simulink model "MORUS_NELINEARNI_NELINEARNI_MPC_2"  (R2019a)
settings: Solver=FixedStepAuto  StartTime=0.0  StopTime=sim_time  RelTol=1e-3  EnableMultiTasking=on
values from neighbouring files (symbols this model uses):
  A_dis_calc = expm(kSamplingTime*A_continous_time)    [MPC_designer_X.m]    (also in NonTilting.m; RUN_simulation.m; Simulacija_MPC_YAW_NELINEARNI.m; Simulacija_MPC_Z.m)
  B_dis_calc = integral_exp_A * B_continous_time    [MPC_designer_X.m]    (also in NonTilting.m; RUN_simulation.m; Simulacija_MPC_YAW_NELINEARNI.m; Simulacija_MPC_Z.m)
  b_f = 4.56e-4    (= 0.000456)    [LinearizacijaMatrica.m]    (also in Linearizirane_matrice.mat; MPC_designer_X.m; NonTilting.m; RUN_simulation.m)
  b_m = 0.01    [LinearizacijaMatrica.m]    (also in Linearizirane_matrice.mat; MPC_designer_X.m; NonTilting.m; RUN_simulation.m)
  BETA = 0.0    (= 0)    [LinearizacijaMatrica.m]    (also in Linearizirane_matrice.mat; MPC_designer_X.m; NonTilting.m = 0.200712863979; RUN_simulation.m)
  g = 9.80665    [LinearizacijaMatrica.m]    (also in Linearizirane_matrice.mat; MPC_designer_X.m = 9.81; NonTilting.m = 9.81; RUN_simulation.m = 9.81)
  hover = 427.6233    [MPC_designer_X.m]    (also in NonTilting.m; RUN_simulation.m; Simulacija_MPC_YAW_NELINEARNI.m; Simulacija_MPC_Z.m)
  I_b_xx = 5.5268    [MPC_designer_X.m]    (also in NonTilting.m; RUN_simulation.m; Simulacija_MPC_YAW_NELINEARNI.m; Simulacija_MPC_Z.m)
  I_b_yy = 5.5268    [MPC_designer_X.m]    (also in NonTilting.m; RUN_simulation.m; Simulacija_MPC_YAW_NELINEARNI.m; Simulacija_MPC_Z.m)
  I_b_zz = 6.8854    [MPC_designer_X.m]    (also in NonTilting.m; RUN_simulation.m; Simulacija_MPC_YAW_NELINEARNI.m; Simulacija_MPC_Z.m)
  kSamplingTime = 0.810    (= 0.81)    [MPCDesigner_YAW.m]    (also in MPC_designer_X.m = 0.1; MPC_designer_Z.m; NonTilting.m = 0.015; RUN_simulation.m = 0.015)
  L = 0.84    [LinearizacijaMatrica.m]    (also in Linearizirane_matrice.mat; MPC_designer_X.m; NonTilting.m; RUN_simulation.m)
  m = 1.0    (= 1)    [LinearizacijaMatrica.m]    (also in Linearizirane_matrice.mat; MPC_designer_X.m; NonTilting.m; RUN_simulation.m)
  M = 34.8    [LinearizacijaMatrica.m]    (also in Linearizirane_matrice.mat; MPC_designer_X.m = 34; NonTilting.m = 34; RUN_simulation.m = 34)
  m_b = 30.8    [LinearizacijaMatrica.m]    (also in Linearizirane_matrice.mat; MPC_designer_X.m; NonTilting.m; RUN_simulation.m)
  odabir = 1    [MPC_designer_X.m]    (also in NonTilting.m; RUN_simulation.m; Simulacija_MPC_YAW_NELINEARNI.m; Simulacija_MPC_Z.m)
  polu = 1.0    (= 1)    [Simulacija_Roll.m]
  Q = inv(diag([0.5800 4*kSamplingTime 0.5800 4*kSamplingTime 300 300 0.2 (0.2/3) 100 4])) * diag([0, 0, 0, 0, 0, 0, 1e5,0, 1e7, 0]) *inv(diag([0.5800 4*kSamplingTime 0.5800 4*kSamplingTime 300 300 0.2 (0.2/3.0) 100 4]))    [NonTilting.m]    (also in RUN_simulation.m = diag([ 0.135340000000000,0.002706800000000,  0.1353400, 0.00; Simulacija_MPC_YAW_NELINEARNI.m = diag([pop(5),pop(6),pop(5),pop(6), pop(7),pop(7),pop(8),pop(; Simulacija_MPC_Z.m = diag([pop(5),pop(6),pop(5),pop(6), pop(7),pop(7),pop(8),pop(; Simulacija_Roll.m = diag([pop(5),pop(6),pop(5),pop(6), pop(7),pop(7),pop(8),pop()
  R = inv(diag([0.5800 0.5800 300 300]))*diag([0, 0, 0, 0])*inv(diag([0.5800 0.5800 300 300]))    [NonTilting.m]    (also in RUN_simulation.m = diag([0.67670, 0.67670, 0.13534000, 0.13534000]); Simulacija_MPC_YAW_NELINEARNI.m = diag([pop(1),pop(1),pop(2),pop(2)]); Simulacija_MPC_Z.m = diag([pop(1),pop(1),pop(2),pop(2)]); Simulacija_Roll.m = diag([pop(1),pop(1),pop(2),pop(2)]))
  R_delta = inv(diag([0.5800 0.5800 300 300]))* diag([0,0,0,0])*inv(diag([0.5800 0.5800 300 300]))    [NonTilting.m]    (also in RUN_simulation.m = diag([0.738879858135067, 0.738879858135067, 0.00738879858135; Simulacija_MPC_YAW_NELINEARNI.m = diag([pop(3),pop(3),pop(4),pop(4)]); Simulacija_MPC_Z.m = diag([pop(3),pop(3),pop(4),pop(4)]); Simulacija_Roll.m = diag([pop(3),pop(3),pop(4),pop(4)]))
  T_r = 0.2    [LinearizacijaMatrica.m]    (also in Linearizirane_matrice.mat; MPC_designer_X.m; NonTilting.m; RUN_simulation.m)
  w_mm = 19.7845    [LinearizacijaMatrica.m]    (also in Linearizirane_matrice.mat; MPC_designer_X.m = 17; NonTilting.m = 17; RUN_simulation.m = 17)
  z_m = 0.05    [LinearizacijaMatrica.m]    (also in Linearizirane_matrice.mat; MPC_designer_X.m; NonTilting.m; RUN_simulation.m)
  z_r = 0.2    [LinearizacijaMatrica.m]    (also in Linearizirane_matrice.mat; MPC_designer_X.m; NonTilting.m; RUN_simulation.m)
  zeta_mm = 0.6544    [LinearizacijaMatrica.m]    (also in Linearizirane_matrice.mat; MPC_designer_X.m = 0.85; NonTilting.m = 0.85; RUN_simulation.m = 0.85)
libraries: simulink x6
(part 2 of 5)

== system MORUS_NELINEARNI_NELINEARNI_MPC_2/REGULATOR Z ==
  Z : Inport
  REF_Z : Inport  Port=2
  DOT_Z : Inport  Port=3
  PID Controller : simulink/Continuous/PID Controller  Controller=PID  Form=Parallel  TimeDomain=Continuous-time  SampleTime=-1  IntegratorMethod=Forward Euler  FilterMethod=Forward Euler  ControllerParametersSource=internal  P=3000.0  I=60.0  D=0.0  UseFilter=on  N=100  TunerSelectOption=Transfer Function Based (PID Tuner App)  InitialConditionSource=internal  InitialConditionForIntegrator=0  InitialConditionForFilter=0  DifferentiatorICPrevScaledInput=0  ExternalReset=none  TrackingMode=off  Kt=1  LimitOutput=off  UpperSaturationLimit=inf  LowerSaturationLimit=-inf  LinearizeAsGain=on  AntiWindupMode=none  Kb=1  POutMin=[]  POutMax=[]  IOutMin=[]  IOutMax=[]  DOutMin=[]  DOutMax=[]  NOutMin=[]  NOutMax=[]  SumOutMin=[]  SumOutMax=[]  SaturationOutMin=[]  SaturationOutMax=[]  PParamMin=[]  PParamMax=[]  IParamMin=[]  IParamMax=[]  DParamMin=[]  DParamMax=[]  NParamMin=[]  NParamMax=[]  KbParamMin=[]  KbParamMax=[]  KtParamMin=[]  KtParamMax=[]  KbOutMin=[]  KbOutMax=[]  KtOutMin=[]  KtOutMax=[]  IntegratorOutMin=[]  IntegratorOutMax=[]  FilterOutMin=[]  FilterOutMax=[]  SumI1OutMin=[]  SumI1OutMax=[]  SumI2OutMin=[]  SumI2OutMax=[]  SumI3OutMin=[]  SumI3OutMax=[]  SumI4OutMin=[]  SumI4OutMax=[]  SumDOutMin=[]  SumDOutMax=[]  DifferentiatorOutMin=[]  DifferentiatorOutMax=[]  FilterDiffOutCoefMin=[]  FilterDiffOutCoefMax=[]  ReciprocalOutMin=[]  ReciprocalOutMax=[]  SumDenOutMin=[]  SumDenOutMax=[]  SumNumOutMin=[]  SumNumOutMax=[]  DivideOutMin=[]  DivideOutMax=[]  IntegratorContinuousStateAttributes=''  IntegratorStateMustResolveToSignalObject=off  IntegratorRTWStateStorageClass=Auto  FilterContinuousStateAttributes=''  FilterStateMustResolveToSignalObject=off  FilterRTWStateStorageClass=Auto  ParallelPVariant=InternalParameters  IdealPVariant=Disabled  IVariant=InternalParameters  DVariant=InternalParameters  IntegratorVariant=Continuous  SatVariant=Disabled  AWVariant=Passthrough  PCopyVariant=Disabled  TRVariant=Disabled  FdbkBlocksVariant=Forward  IdealPFdbkVariant=Disabled  SatFdbkVariant=Disabled  DerivativeFilterVariant=ContFilter  NVariant=InternalParameters  NCopyVariant=Disabled  FilterICVariant=InternalICsFilter  IntegratorICVariant=InternalICs  ExternalResetVariant=Disabled  TRSumVariant=Passthrough  SumFdbkVariant=Disabled  SumVariant=Sum_PID
  PID Controller1 : simulink/Continuous/PID Controller  Controller=PID  Form=Parallel  TimeDomain=Continuous-time  SampleTime=-1  IntegratorMethod=Forward Euler  FilterMethod=Forward Euler  ControllerParametersSource=internal  P=4.1  I=0.1  D=0  UseFilter=on  N=100  TunerSelectOption=Transfer Function Based (PID Tuner App)  InitialConditionSource=internal  InitialConditionForIntegrator=0  InitialConditionForFilter=0  DifferentiatorICPrevScaledInput=0  ExternalReset=none  TrackingMode=off  Kt=1  LimitOutput=off  UpperSaturationLimit=inf  LowerSaturationLimit=-inf  LinearizeAsGain=on  AntiWindupMode=none  Kb=1  POutMin=[]  POutMax=[]  IOutMin=[]  IOutMax=[]  DOutMin=[]  DOutMax=[]  NOutMin=[]  NOutMax=[]  SumOutMin=[]  SumOutMax=[]  SaturationOutMin=[]  SaturationOutMax=[]  PParamMin=[]  PParamMax=[]  IParamMin=[]  IParamMax=[]  DParamMin=[]  DParamMax=[]  NParamMin=[]  NParamMax=[]  KbParamMin=[]  KbParamMax=[]  KtParamMin=[]  KtParamMax=[]  KbOutMin=[]  KbOutMax=[]  KtOutMin=[]  KtOutMax=[]  IntegratorOutMin=[]  IntegratorOutMax=[]  FilterOutMin=[]  FilterOutMax=[]  SumI1OutMin=[]  SumI1OutMax=[]  SumI2OutMin=[]  SumI2OutMax=[]  SumI3OutMin=[]  SumI3OutMax=[]  SumI4OutMin=[]  SumI4OutMax=[]  SumDOutMin=[]  SumDOutMax=[]  DifferentiatorOutMin=[]  DifferentiatorOutMax=[]  FilterDiffOutCoefMin=[]  FilterDiffOutCoefMax=[]  ReciprocalOutMin=[]  ReciprocalOutMax=[]  SumDenOutMin=[]  SumDenOutMax=[]  SumNumOutMin=[]  SumNumOutMax=[]  DivideOutMin=[]  DivideOutMax=[]  IntegratorContinuousStateAttributes=''  IntegratorStateMustResolveToSignalObject=off  IntegratorRTWStateStorageClass=Auto  FilterContinuousStateAttributes=''  FilterStateMustResolveToSignalObject=off  FilterRTWStateStorageClass=Auto  ParallelPVariant=InternalParameters  IdealPVariant=Disabled  IVariant=InternalParameters  DVariant=InternalParameters  IntegratorVariant=Continuous  SatVariant=Disabled  AWVariant=Passthrough  PCopyVariant=Disabled  TRVariant=Disabled  FdbkBlocksVariant=Forward  IdealPFdbkVariant=Disabled  SatFdbkVariant=Disabled  DerivativeFilterVariant=ContFilter  NVariant=InternalParameters  NCopyVariant=Disabled  FilterICVariant=InternalICsFilter  IntegratorICVariant=InternalICs  ExternalResetVariant=Disabled  TRSumVariant=Passthrough  SumFdbkVariant=Disabled  SumVariant=Sum_PID
  Scope : Scope
  Scope1 : Scope
  Sum : Sum  Inputs=|+-
  Sum1 : Sum  Inputs=|+-
  SIGNAL_Z : Outport
  wires:
  REF_Z/1 -> Sum/1
  Z/1 -> Sum/2, Scope1/1
  Sum1/1 -> Scope/1, PID Controller/1  "Error"
  PID Controller1/1 -> Sum1/1
  Sum/1 -> PID Controller1/1
  DOT_Z/1 -> Sum1/2
  PID Controller/1 -> SIGNAL_Z/1

== system MORUS_NELINEARNI_NELINEARNI_MPC_2/ROLL SATURATION SIGNAL ==
  In1 : Inport
  In2 : Inport  Port=2
  In3 : Inport  Port=3
  In4 : Inport  Port=4
  Gain{1..3,5} (4 alike) : Gain  Gain=-1
  Mux2 : Mux
  ROLL_SATURATION_SIGNAL : Outport
  wires:
  Mux2/1 -> ROLL_SATURATION_SIGNAL/1  "PropSpeedCmd"
  Gain5/1 -> Mux2/1
  Gain1/1 -> Mux2/2
  Gain2/1 -> Mux2/3
  Gain3/1 -> Mux2/4
  In4/1 -> Gain3/1
  In3/1 -> Gain2/1
  In2/1 -> Gain1/1
  In1/1 -> Gain5/1

== system MORUS_NELINEARNI_NELINEARNI_MPC_2/ROLL_SATURATION_STATE_SPACE ==
  hover : Inport
  REF_ROLL : Inport  Port=2
  In1 : Inport  Port=3
  In2 : Inport  Port=4
  In3 : Inport  Port=5
  In4 : Inport  Port=6
  In5 : Inport  Port=7
  In6 : Inport  Port=8
  In7 : Inport  Port=9
  In8 : Inport  Port=10
  Gain{,1..3} (4 alike) : Gain  Gain=-1
  Mux2 : Mux  Inputs=8
  Scope : Scope
  Scope1 : Scope
  Sum : Sum  Inputs=|+-
  Sum1 : Sum  Inputs=|+-
  Sum2 : Sum  Inputs=|+-
  ROLL_X_SS : Outport
  wires:
  Mux2/1 -> ROLL_X_SS/1  "PropSpeedCmd"
  REF_ROLL/1 -> Sum/1
  Sum/1 -> Scope1/1, Mux2/7
  Sum2/1 -> Mux2/5
  Sum1/1 -> Mux2/6
  hover/1 -> Sum1/1, Sum2/1
  In1/1 -> Gain/1
  Gain/1 -> Mux2/1
  In2/1 -> Gain1/1
  Gain1/1 -> Mux2/2
  In3/1 -> Gain2/1
  Gain2/1 -> Mux2/3
  In4/1 -> Gain3/1
  Gain3/1 -> Mux2/4
  In5/1 -> Sum2/2
  In6/1 -> Sum1/2
  In7/1 -> Scope/1, Sum/2
  In8/1 -> Mux2/8

== system MORUS_NELINEARNI_NELINEARNI_MPC_2/ROLL_STATE_SPACE ==
  y_2 : Inport
  DOT_y_2 : Inport  Port=2
  y_4 : Inport  Port=3
  DOT_y_4 : Inport  Port=4
  ROTOR_2 : Inport  Port=5
  ROTOR_4 : Inport  Port=6
  ROLL : Inport  Port=7
  DOT_ROLL : Inport  Port=8
  hover : Inport  Port=9
  Gain{,1..3} (4 alike) : Gain  Gain=-1
  Gain{4..12} (9 alike) : Gain  Gain=0
  Mux : Mux  Inputs=8
  Sum : Sum  Inputs=|+-
  Sum1 : Sum  Inputs=|+-
  ROLL_STATE_SPACE : Outport
  wires:
  Mux/1 -> ROLL_STATE_SPACE/1
  y_2/1 -> Gain12/1
  DOT_y_2/1 -> Gain11/1
  y_4/1 -> Gain10/1
  DOT_y_4/1 -> Gain9/1
  ROLL/1 -> Gain6/1
  DOT_ROLL/1 -> Gain5/1
  ROTOR_2/1 -> Sum/1
  ROTOR_4/1 -> Sum1/1
  hover/1 -> Gain4/1
  Gain/1 -> Mux/1
  Gain1/1 -> Mux/2
  Gain2/1 -> Mux/3
  Gain3/1 -> Mux/4
  Sum/1 -> Gain8/1
  Sum1/1 -> Gain7/1
  Gain4/1 -> Sum/2, Sum1/2
  Gain5/1 -> Mux/8
  Gain6/1 -> Mux/7
  Gain7/1 -> Mux/6
  Gain8/1 -> Mux/5
  Gain9/1 -> Gain3/1
  Gain10/1 -> Gain2/1
  Gain11/1 -> Gain1/1
  Gain12/1 -> Gain/1

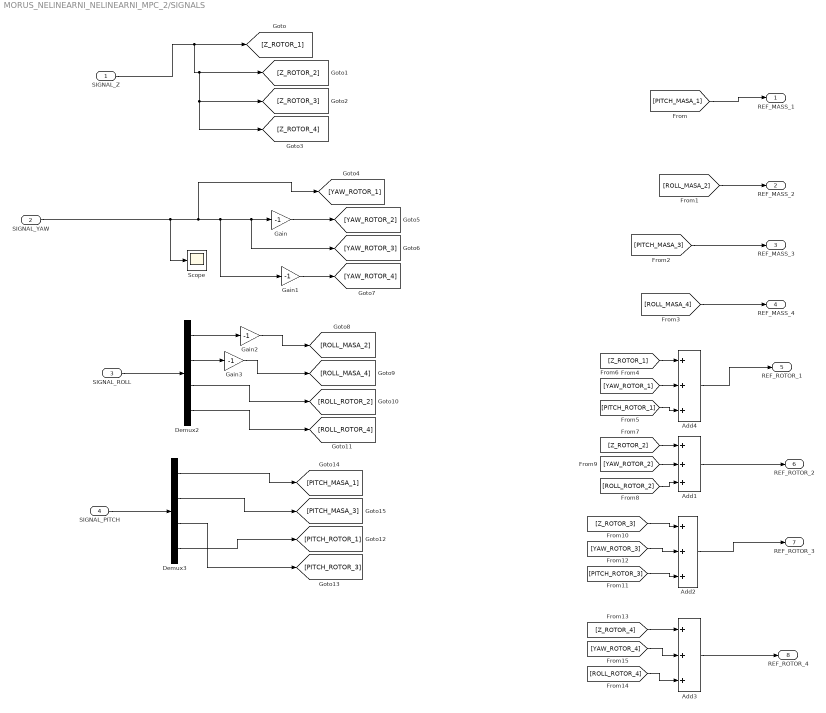
== system MORUS_NELINEARNI_NELINEARNI_MPC_2/SIGNALS ==
  SIGNAL_Z : Inport
  SIGNAL_YAW : Inport  Port=2
  SIGNAL_ROLL : Inport  Port=3
  SIGNAL_PITCH : Inport  Port=4
  Add{1..4} (4 alike) : Sum  Inputs=+++  AccumDataTypeStr=double  OutDataTypeStr=double
  Demux2 : Demux
  Demux3 : Demux
  Gain{,1..3} (4 alike) : Gain  Gain=-1
  Scope : Scope
  REF_MASS_1 : Outport
  REF_MASS_2 : Outport  Port=2
  REF_MASS_3 : Outport  Port=3
  REF_MASS_4 : Outport  Port=4
  REF_ROTOR_1 : Outport  Port=5
  REF_ROTOR_2 : Outport  Port=6
  REF_ROTOR_3 : Outport  Port=7
  REF_ROTOR_4 : Outport  Port=8
  wires:
  [PITCH_MASA_1] -> REF_MASS_1/1
  [ROLL_MASA_2] -> REF_MASS_2/1
  [PITCH_MASA_3] -> REF_MASS_3/1
  [ROLL_MASA_4] -> REF_MASS_4/1
  Add4/1 -> REF_ROTOR_1/1
  Add1/1 -> REF_ROTOR_2/1
  Add2/1 -> REF_ROTOR_3/1
  Add3/1 -> REF_ROTOR_4/1
  SIGNAL_Z/1 -> [Z_ROTOR_4], [Z_ROTOR_3], [Z_ROTOR_2], [Z_ROTOR_1]
  SIGNAL_ROLL/1 -> Demux2/1
  Demux2/1 -> Gain2/1
  Demux2/2 -> Gain3/1
  Demux3/1 -> [PITCH_MASA_1]
  Demux3/4 -> [PITCH_ROTOR_1]
  Demux3/2 -> [PITCH_MASA_3]
  Demux3/3 -> [PITCH_ROTOR_3]
  SIGNAL_PITCH/1 -> Demux3/1
  [Z_ROTOR_1] -> Add4/1
  [YAW_ROTOR_1] -> Add4/2
  [PITCH_ROTOR_1] -> Add4/3
  [Z_ROTOR_2] -> Add1/1
  [ROLL_ROTOR_2] -> Add1/3
  [YAW_ROTOR_2] -> Add1/2
  [Z_ROTOR_3] -> Add2/1
  [YAW_ROTOR_3] -> Add2/2
  [PITCH_ROTOR_3] -> Add2/3
  [Z_ROTOR_4] -> Add3/1
  [YAW_ROTOR_4] -> Add3/2
  [ROLL_ROTOR_4] -> Add3/3
  Gain/1 -> [YAW_ROTOR_2]
  Gain1/1 -> [YAW_ROTOR_4]
  Gain2/1 -> [ROLL_MASA_2]
  Gain3/1 -> [ROLL_MASA_4]
  Demux2/4 -> [ROLL_ROTOR_4]
  Demux2/3 -> [ROLL_ROTOR_2]
  SIGNAL_YAW/1 -> Scope/1, [YAW_ROTOR_1], Gain1/1, [YAW_ROTOR_3], Gain/1

== system MORUS_NELINEARNI_NELINEARNI_MPC_2/Subsystem ==
  AUTO_REF_MASS_1 : Inport
  AUTO_REF_MASS_2 : Inport  Port=2
  AUTO_REF_MASS_3 : Inport  Port=3
  AUTO_REF_MASS_4 : Inport  Port=4
  AUTO_REF_ROTOR_1 : Inport  Port=5
  AUTO_REF_ROTOR_2 : Inport  Port=6
  AUTO_REF_ROTOR_3 : Inport  Port=7
  AUTO_REF_ROTOR_4 : Inport  Port=8
  MANUAL_SIGNAL : Inport  Port=9
  MANUAL_REF_MASS_1 : Inport  Port=10
  MANUAL_REF_MASS_2 : Inport  Port=11
  MANUAL_REF_MASS_3 : Inport  Port=12
  MANUAL_REF_MASS_4 : Inport  Port=13
  MANUAL_REF_ROTOR_1 : Inport  Port=14
  MANUAL_REF_ROTOR_2 : Inport  Port=15
  MANUAL_REF_ROTOR_3 : Inport  Port=16
  MANUAL_REF_ROTOR_4 : Inport  Port=17
  Switch{,1..7} (8 alike) : Switch  Criteria=u2 > Threshold
  REF_MASS_1 : Outport
  REF_MASS_2 : Outport  Port=2
  REF_MASS_3 : Outport  Port=3
  REF_MASS_4 : Outport  Port=4
  REF_ROTOR_1 : Outport  Port=5
  REF_ROTOR_2 : Outport  Port=6
  REF_ROTOR_3 : Outport  Port=7
  REF_ROTOR_4 : Outport  Port=8
  wires:
  AUTO_REF_MASS_1/1 -> Switch/3
  AUTO_REF_MASS_2/1 -> Switch1/3
  AUTO_REF_MASS_3/1 -> Switch2/3
  AUTO_REF_MASS_4/1 -> Switch3/3
  AUTO_REF_ROTOR_1/1 -> Switch4/3
  AUTO_REF_ROTOR_2/1 -> Switch5/3
  AUTO_REF_ROTOR_3/1 -> Switch6/3
  AUTO_REF_ROTOR_4/1 -> Switch7/3
  MANUAL_SIGNAL/1 -> Switch6/2, Switch7/2, Switch5/2, Switch1/2, Switch/2, Switch2/2, Switch4/2, Switch3/2
  Switch7/1 -> REF_ROTOR_4/1
  Switch6/1 -> REF_ROTOR_3/1
  Switch5/1 -> REF_ROTOR_2/1
  Switch4/1 -> REF_ROTOR_1/1
  Switch3/1 -> REF_MASS_4/1
  Switch2/1 -> REF_MASS_3/1
  Switch1/1 -> REF_MASS_2/1
  Switch/1 -> REF_MASS_1/1
  MANUAL_REF_MASS_1/1 -> Switch/1
  MANUAL_REF_MASS_2/1 -> Switch1/1
  MANUAL_REF_MASS_3/1 -> Switch2/1
  MANUAL_REF_MASS_4/1 -> Switch3/1
  MANUAL_REF_ROTOR_1/1 -> Switch4/1
  MANUAL_REF_ROTOR_2/1 -> Switch5/1
  MANUAL_REF_ROTOR_3/1 -> Switch6/1
  MANUAL_REF_ROTOR_4/1 -> Switch7/1

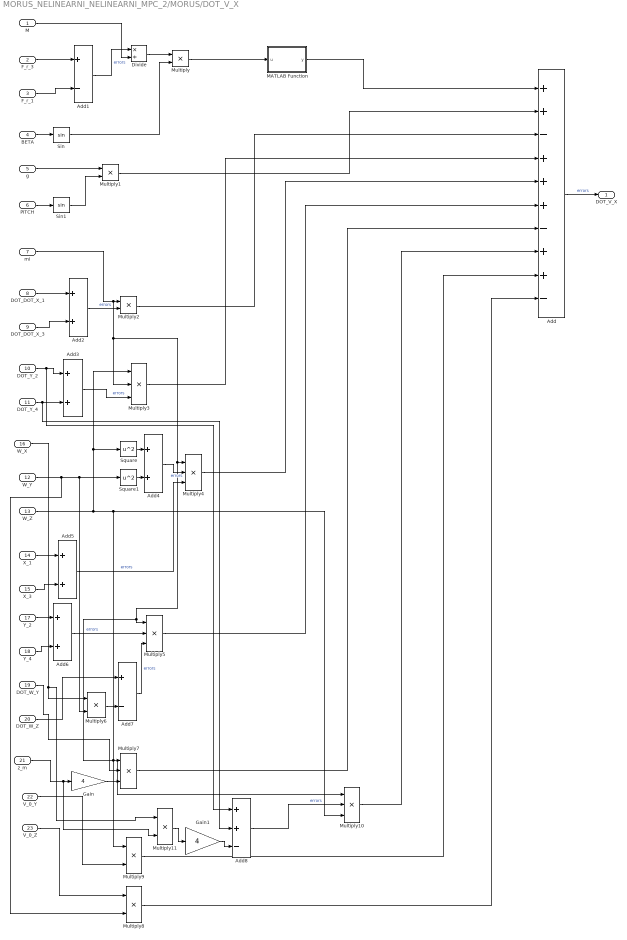
== system MORUS_NELINEARNI_NELINEARNI_MPC_2/MORUS/DOT_V_X ==
  M : Inport
  F_r_3 : Inport  Port=2
  F_r_1 : Inport  Port=3
  BETA : Inport  Port=4
  g : Inport  Port=5
  PITCH : Inport  Port=6
  mi : Inport  Port=7
  DOT_DOT_X_1 : Inport  Port=8
  DOT_DOT_X_3 : Inport  Port=9
  DOT_Y_2 : Inport  Port=10
  DOT_Y_4 : Inport  Port=11
  W_Y : Inport  Port=12
  W_Z : Inport  Port=13
  X_1 : Inport  Port=14
  X_3 : Inport  Port=15
  W_X : Inport  Port=16
  Y_2 : Inport  Port=17
  Y_4 : Inport  Port=18
  DOT_W_Y : Inport  Port=19
  DOT_W_Z : Inport  Port=20
  z_m : Inport  Port=21
  V_0_Y : Inport  Port=22
  V_0_Z : Inport  Port=23
  Add : Sum  Inputs=++-+++-++-  AccumDataTypeStr=double  OutDataTypeStr=double
  Add1 : Sum  Inputs=+-  AccumDataTypeStr=double  OutDataTypeStr=double
  Add{2..6} (5 alike) : Sum  AccumDataTypeStr=double  OutDataTypeStr=double
  Add7 : Sum  Inputs=+-  AccumDataTypeStr=double  OutDataTypeStr=double
  Add8 : Sum  Inputs=++-  AccumDataTypeStr=double  OutDataTypeStr=double
  Divide : Product  Inputs=*/
  Gain : Gain  Gain=4
  Gain1 : Gain  Gain=4
  MATLAB Function : MATLAB Function  TreatAsAtomicUnit=on
  Multiply{,1..2,6,8..9,11} (7 alike) : Product
  Multiply{3..5,7,10} (5 alike) : Product  Inputs=3
  Sin : Trigonometry
  Sin1 : Trigonometry
  Square : Math  Operator=square  OutDataTypeStr=double  SaturateOnIntegerOverflow=on
  Square1 : Math  Operator=square  OutDataTypeStr=double  SaturateOnIntegerOverflow=on
  DOT_V_X : Outport
  wires:
  Add/1 -> DOT_V_X/1  "errors"
  F_r_3/1 -> Add1/1
  F_r_1/1 -> Add1/2
  Divide/1 -> Multiply/1
  BETA/1 -> Sin/1
  Sin/1 -> Multiply/2
  Multiply/1 -> MATLAB Function/1(u)
  g/1 -> Multiply1/1
  PITCH/1 -> Sin1/1
  Sin1/1 -> Multiply1/2
  Multiply1/1 -> Add/2
  DOT_DOT_X_1/1 -> Add2/1
  DOT_DOT_X_3/1 -> Add2/2
  Add2/1 -> Multiply2/2  "errors"
  mi/1 -> Multiply3/2, Multiply10/1, Multiply7/1, Multiply5/1, Multiply4/1, Multiply2/1
  Multiply2/1 -> Add/3
  DOT_Y_2/1 -> Add8/1, Add3/1
  DOT_Y_4/1 -> Add8/2, Add3/2
  Add3/1 -> Multiply3/3  "errors"
  W_Z/1 -> Multiply9/1, Multiply10/3, Square/1, Multiply3/1
  Multiply3/1 -> Add/4
  W_Y/1 -> Multiply8/2, Multiply6/2, Square1/1
  Square1/1 -> Add4/2
  Square/1 -> Add4/1
  Add4/1 -> Multiply4/2  "errors"
  X_1/1 -> Add5/1
  X_3/1 -> Add5/2
  Add5/1 -> Multiply4/3  "errors"
  Multiply4/1 -> Add/5
  Y_2/1 -> Add6/1
  Y_4/1 -> Add6/2
  Add6/1 -> Multiply5/2  "errors"
  Multiply6/1 -> Add7/2
  DOT_W_Z/1 -> Add7/1
  Add7/1 -> Multiply5/3  "errors"
  W_X/1 -> Multiply11/1, Multiply6/1
  Multiply5/1 -> Add/6
  Gain/1 -> Multiply7/3
  z_m/1 -> Multiply11/2, Gain/1
  DOT_W_Y/1 -> Multiply7/2
  Multiply7/1 -> Add/7
  V_0_Y/1 -> Multiply9/2
  Multiply9/1 -> Add/9
  V_0_Z/1 -> Multiply8/1
  Multiply8/1 -> Add/10
  Add8/1 -> Multiply10/2  "errors"
  Gain1/1 -> Add8/3
  Multiply11/1 -> Gain1/1
  Multiply10/1 -> Add/8
  MATLAB Function/1(y) -> Add/1
  Add1/1 -> Divide/1  "errors"
  M/1 -> Divide/2

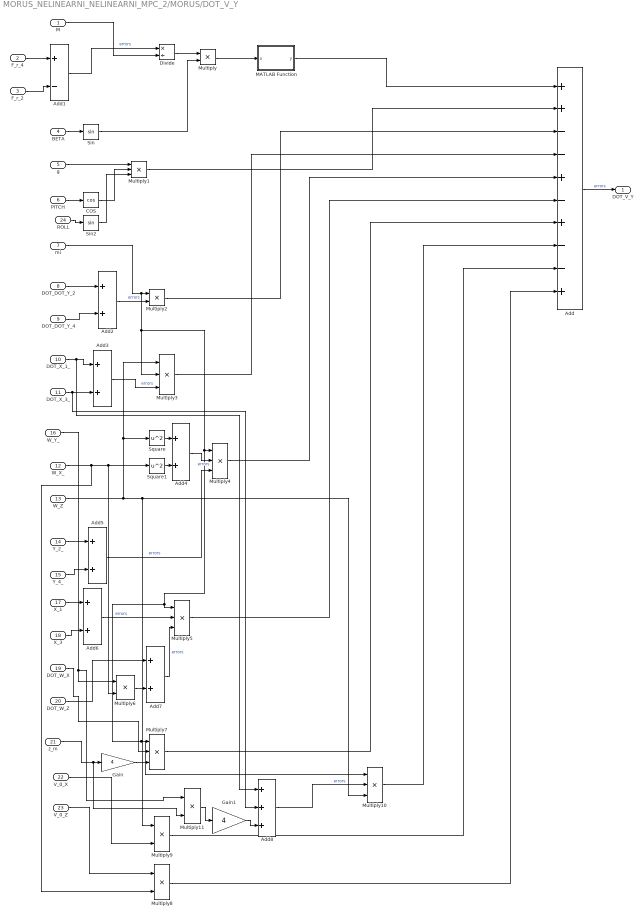
== system MORUS_NELINEARNI_NELINEARNI_MPC_2/MORUS/DOT_V_Y ==
  M : Inport
  F_r_4 : Inport  Port=2
  F_r_2 : Inport  Port=3
  BETA : Inport  Port=4
  g : Inport  Port=5
  PITCH : Inport  Port=6
  mi : Inport  Port=7
  DOT_DOT_Y_2 : Inport  Port=8
  DOT_DOT_Y_4 : Inport  Port=9
  DOT_X_1_ : Inport  Port=10
  DOT_X_3_ : Inport  Port=11
  W_X_ : Inport  Port=12
  W_Z : Inport  Port=13
  Y_2_ : Inport  Port=14
  Y_4_ : Inport  Port=15
  W_Y_ : Inport  Port=16
  X_1 : Inport  Port=17
  X_3 : Inport  Port=18
  DOT_W_X : Inport  Port=19
  DOT_W_Z : Inport  Port=20
  z_m : Inport  Port=21
  V_0_X : Inport  Port=22
  V_0_Z : Inport  Port=23
  ROLL : Inport  Port=24
  Add : Sum  Inputs=++--+-+--+  AccumDataTypeStr=double  OutDataTypeStr=double
  Add1 : Sum  Inputs=+-  AccumDataTypeStr=double  OutDataTypeStr=double
  Add{2..7} (6 alike) : Sum  AccumDataTypeStr=double  OutDataTypeStr=double
  Add8 : Sum  Inputs=+++  AccumDataTypeStr=double  OutDataTypeStr=double
  COS : Trigonometry  Operator=cos
  Divide : Product  Inputs=*/
  Gain : Gain  Gain=4
  Gain1 : Gain  Gain=4
  MATLAB Function : MATLAB Function  TreatAsAtomicUnit=on
  Multiply{,2,6,8..9,11} (6 alike) : Product
  Multiply{1,3..5,7,10} (6 alike) : Product  Inputs=3
  Sin : Trigonometry
  Sin2 : Trigonometry
  Square : Math  Operator=square  SaturateOnIntegerOverflow=on
  Square1 : Math  Operator=square  SaturateOnIntegerOverflow=on
  DOT_V_Y : Outport
  wires:
  Add/1 -> DOT_V_Y/1  "errors"
  F_r_4/1 -> Add1/1
  F_r_2/1 -> Add1/2
  Divide/1 -> Multiply/1
  BETA/1 -> Sin/1
  Sin/1 -> Multiply/2
  g/1 -> Multiply1/1
  PITCH/1 -> COS/1
  COS/1 -> Multiply1/2
  Multiply1/1 -> Add/2
  DOT_DOT_Y_2/1 -> Add2/1
  DOT_DOT_Y_4/1 -> Add2/2
  Add2/1 -> Multiply2/2  "errors"
  mi/1 -> Multiply3/2, Multiply10/1, Multiply7/1, Multiply5/1, Multiply4/1, Multiply2/1
  Multiply2/1 -> Add/3
  DOT_X_1_/1 -> Add8/1, Add3/1
  DOT_X_3_/1 -> Add8/2, Add3/2
  Add3/1 -> Multiply3/3  "errors"
  W_Z/1 -> Multiply9/1, Multiply10/3, Square/1, Multiply3/1
  Multiply3/1 -> Add/4
  W_X_/1 -> Multiply8/2, Multiply6/2, Square1/1
  Square1/1 -> Add4/2
  Square/1 -> Add4/1
  Add4/1 -> Multiply4/2  "errors"
  Y_2_/1 -> Add5/1
  Y_4_/1 -> Add5/2
  Add5/1 -> Multiply4/3  "errors"
  Multiply4/1 -> Add/5
  X_1/1 -> Add6/1
  X_3/1 -> Add6/2
  Add6/1 -> Multiply5/2  "errors"
  Multiply6/1 -> Add7/2
  DOT_W_Z/1 -> Add7/1
  Add7/1 -> Multiply5/3  "errors"
  W_Y_/1 -> Multiply11/1, Multiply6/1
  Multiply5/1 -> Add/6
  Gain/1 -> Multiply7/3
  z_m/1 -> Multiply11/2, Gain/1
  DOT_W_X/1 -> Multiply7/2
  Multiply7/1 -> Add/7
  V_0_X/1 -> Multiply9/2
  Multiply9/1 -> Add/9
  V_0_Z/1 -> Multiply8/1
  Multiply8/1 -> Add/10
  Add8/1 -> Multiply10/2  "errors"
  Gain1/1 -> Add8/3
  Multiply11/1 -> Gain1/1
  Multiply10/1 -> Add/8
  ROLL/1 -> Sin2/1
  Sin2/1 -> Multiply1/3
  Multiply/1 -> MATLAB Function/1(u)
  MATLAB Function/1(y) -> Add/1
  M/1 -> Divide/2
  Add1/1 -> Divide/1  "errors"

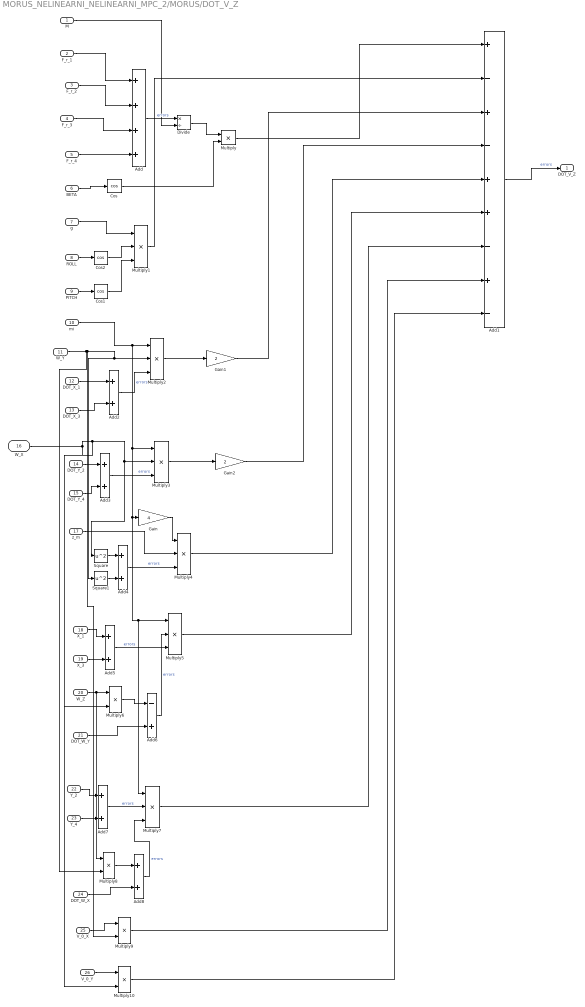
== system MORUS_NELINEARNI_NELINEARNI_MPC_2/MORUS/DOT_V_Z ==
  M : Inport
  F_r_1 : Inport  Port=2
  F_r_2 : Inport  Port=3
  F_r_3 : Inport  Port=4
  F_r_4 : Inport  Port=5
  BETA : Inport  Port=6
  g : Inport  Port=7
  ROLL : Inport  Port=8
  PITCH : Inport  Port=9
  mi : Inport  Port=10
  W_Y : Inport  Port=11
  DOT_X_1 : Inport  Port=12
  DOT_X_3 : Inport  Port=13
  DOT_Y_2 : Inport  Port=14
  DOT_Y_4 : Inport  Port=15
  W_X : Inport  Port=16
  z_m : Inport  Port=17
  X_1 : Inport  Port=18
  X_3 : Inport  Port=19
  W_Z : Inport  Port=20
  DOT_W_Y : Inport  Port=21
  Y_2 : Inport  Port=22
  Y_4 : Inport  Port=23
  DOT_W_X : Inport  Port=24
  V_0_X : Inport  Port=25
  V_0_Y : Inport  Port=26
  Add : Sum  Inputs=++++  AccumDataTypeStr=double  OutDataTypeStr=double
  Add1 : Sum  Inputs=+-+-++-+-  AccumDataTypeStr=double  OutDataTypeStr=double
  Add{2..5,7..8} (6 alike) : Sum  AccumDataTypeStr=double  OutDataTypeStr=double
  Add6 : Sum  Inputs=-+  AccumDataTypeStr=double  OutDataTypeStr=double
  Cos : Trigonometry  Operator=cos
  Cos1 : Trigonometry  Operator=cos
  Cos2 : Trigonometry  Operator=cos
  Divide : Product  Inputs=*/
  Gain : Gain  Gain=4
  Gain1 : Gain  Gain=2
  Gain2 : Gain  Gain=2
  Multiply{,6,8..10} (5 alike) : Product
  Multiply{1..5,7} (6 alike) : Product  Inputs=3
  Square : Math  Operator=square  SaturateOnIntegerOverflow=on
  Square1 : Math  Operator=square  SaturateOnIntegerOverflow=on
  DOT_V_Z : Outport
  wires:
  F_r_1/1 -> Add/1
  F_r_2/1 -> Add/2
  F_r_3/1 -> Add/3
  F_r_4/1 -> Add/4
  Add/1 -> Divide/1  "errors"
  M/1 -> Divide/2
  BETA/1 -> Cos/1
  Divide/1 -> Multiply/1
  Cos/1 -> Multiply/2
  Add1/1 -> DOT_V_Z/1  "errors"
  Multiply/1 -> Add1/1
  PITCH/1 -> Cos1/1
  ROLL/1 -> Cos2/1
  g/1 -> Multiply1/1
  Cos2/1 -> Multiply1/2
  Cos1/1 -> Multiply1/3
  Multiply1/1 -> Add1/2
  DOT_X_1/1 -> Add2/1
  DOT_X_3/1 -> Add2/2
  mi/1 -> Multiply3/1, Multiply7/1, Multiply5/1, Gain/1, Multiply2/1
  W_Y/1 -> Multiply9/2, Square1/1, Multiply2/2, Multiply8/2
  Add2/1 -> Multiply2/3  "errors"
  Multiply2/1 -> Gain1/1
  DOT_Y_4/1 -> Add3/2
  DOT_Y_2/1 -> Add3/1
  Add3/1 -> Multiply3/3  "errors"
  W_X/1 -> Multiply6/2, Square/1, Multiply3/2, Multiply10/2
  Multiply3/1 -> Gain2/1
  Square/1 -> Add4/1
  Square1/1 -> Add4/2
  Add4/1 -> Multiply4/3  "errors"
  z_m/1 -> Multiply4/2
  Gain/1 -> Multiply4/1
  Multiply4/1 -> Add1/5
  X_1/1 -> Add5/1
  X_3/1 -> Add5/2
  Add5/1 -> Multiply5/3  "errors"
  W_Z/1 -> Multiply8/1, Multiply6/1
  Multiply6/1 -> Add6/1
  Add6/1 -> Multiply5/2  "errors"
  DOT_W_Y/1 -> Add6/2
  Multiply5/1 -> Add1/6
  Y_2/1 -> Add7/1
  Y_4/1 -> Add7/2
  Add7/1 -> Multiply7/2  "errors"
  DOT_W_X/1 -> Add8/2
  Multiply8/1 -> Add8/1
  Add8/1 -> Multiply7/3  "errors"
  Multiply7/1 -> Add1/7
  Gain1/1 -> Add1/3
  Gain2/1 -> Add1/4
  V_0_Y/1 -> Multiply10/1
  V_0_X/1 -> Multiply9/1
  Multiply9/1 -> Add1/8
  Multiply10/1 -> Add1/9

== system MORUS_NELINEARNI_NELINEARNI_MPC_2/MORUS/Force rotor 1 ==
  rotor_1 : Inport
  b_f : Inport  Port=2
  Multiply : Product  OutDataTypeStr=double
  Square : Math  Operator=square  OutDataTypeStr=double  SaturateOnIntegerOverflow=on
  Force_1 : Outport
  wires:
  Multiply/1 -> Force_1/1
  b_f/1 -> Multiply/2
  rotor_1/1 -> Square/1
  Square/1 -> Multiply/1

== system MORUS_NELINEARNI_NELINEARNI_MPC_2/MORUS/Force rotor 2 ==
  rotor_2 : Inport
  b_f : Inport  Port=2
  Multiply : Product  OutDataTypeStr=double
  Square : Math  Operator=square  OutDataTypeStr=double  SaturateOnIntegerOverflow=on
  Force_2 : Outport
  wires:
  Multiply/1 -> Force_2/1
  b_f/1 -> Multiply/2
  rotor_2/1 -> Square/1
  Square/1 -> Multiply/1

== system MORUS_NELINEARNI_NELINEARNI_MPC_2/MORUS/Force rotor 3 ==
  rotor_3 : Inport
  b_f : Inport  Port=2
  Multiply : Product  OutDataTypeStr=double
  Square : Math  Operator=square  OutDataTypeStr=double  SaturateOnIntegerOverflow=on
  Force_3 : Outport
  wires:
  Multiply/1 -> Force_3/1
  b_f/1 -> Multiply/2
  rotor_3/1 -> Square/1
  Square/1 -> Multiply/1

== system MORUS_NELINEARNI_NELINEARNI_MPC_2/MORUS/Force rotor 4 ==
  rotor_4 : Inport
  b_f : Inport  Port=2
  Multiply : Product  OutDataTypeStr=double
  Square : Math  Operator=square  OutDataTypeStr=double  SaturateOnIntegerOverflow=on
  Force_4 : Outport
  wires:
  Multiply/1 -> Force_4/1
  b_f/1 -> Multiply/2
  rotor_4/1 -> Square/1
  Square/1 -> Multiply/1

== system MORUS_NELINEARNI_NELINEARNI_MPC_2/MORUS/ICE ROTOR 2 ==
  ref_rotor_2 : Inport
  Transfer Fcn : TransferFcn  Denominator=[T_r 1]
  rotor_2 : Outport
  wires:
  ref_rotor_2/1 -> Transfer Fcn/1
  Transfer Fcn/1 -> rotor_2/1

== system MORUS_NELINEARNI_NELINEARNI_MPC_2/MORUS/ICE ROTOR 3 ==
  ref_rotor_3 : Inport
  Transfer Fcn : TransferFcn  Denominator=[T_r 1]
  rotor_3 : Outport
  wires:
  ref_rotor_3/1 -> Transfer Fcn/1
  Transfer Fcn/1 -> rotor_3/1

== system MORUS_NELINEARNI_NELINEARNI_MPC_2/MORUS/ICE ROTOR 4 ==
  ref_rotor_4 : Inport
  Transfer Fcn : TransferFcn  Denominator=[T_r 1]
  rotor_4 : Outport
  wires:
  ref_rotor_4/1 -> Transfer Fcn/1
  Transfer Fcn/1 -> rotor_4/1

== system MORUS_NELINEARNI_NELINEARNI_MPC_2/MORUS/ICE(Internal combustion engine) ROTOR 1 ==
  ref_rotor_1 : Inport
  Transfer Fcn : TransferFcn  Denominator=[T_r 1]
  rotor_1 : Outport
  wires:
  ref_rotor_1/1 -> Transfer Fcn/1
  Transfer Fcn/1 -> rotor_1/1

== system MORUS_NELINEARNI_NELINEARNI_MPC_2/MORUS/I_1_c ==
  m : Inport
  mi : Inport  Port=2
  z_m : Inport  Port=3
  y2 : Inport  Port=4
  y4 : Inport  Port=5
  x1 : Inport  Port=6
  x3 : Inport  Port=7
  L : Inport  Port=8
  I_11 : Subsystem
  I_12 / I_21 : Subsystem
  I_13 / I_31 : Subsystem
  I_22 : Subsystem
  I_23 / I_32 : Subsystem
  I_33 : Subsystem
  Mux : Mux  Inputs=9
  I_1_c : Outport
  wires:
  I_11/1(I_11) -> Mux/1
  I_12 / I_21/1(I_12) -> Mux/2, Mux/4
  I_13 / I_31/1(I_13) -> Mux/3, Mux/7
  I_22/1(I_22) -> Mux/5
  I_23 / I_32/1(I_23) -> Mux/6, Mux/8
  I_33/1(I_33) -> Mux/9
  Mux/1 -> I_1_c/1  "PropSpeedCmd"
  m/1 -> I_12 / I_21/1(m), I_33/3(m), I_23 / I_32/1(m), I_22/3(m), I_13 / I_31/1(m), I_11/3(m)
  mi/1 -> I_33/4(mi), I_23 / I_32/2(mi), I_22/4(mi), I_13 / I_31/2(mi), I_12 / I_21/2(mi), I_11/4(mi)
  y2/1 -> I_33/6(y2), I_23 / I_32/3(y_2), I_11/1(y2), I_12 / I_21/5(y_2)
  L/1 -> I_12 / I_21/7(L), I_22/6(L), I_13 / I_31/5(L), I_33/5(L)
  z_m/1 -> I_23 / I_32/5(z_m), I_13 / I_31/6(z_m), I_22/5(z_m), I_11/5(z_m)
  x1/1 -> I_22/1(x1), I_33/1(x1), I_13 / I_31/3(x_1), I_12 / I_21/3(x_1)
  x3/1 -> I_13 / I_31/4(x_3), I_12 / I_21/4(x_3), I_22/2(x3), I_33/2(x3)
  y4/1 -> I_33/7(y4), I_23 / I_32/4(y_4), I_11/2(y4), I_12 / I_21/6(y_4)

== system MORUS_NELINEARNI_NELINEARNI_MPC_2/MORUS/I_2_c ==
  m : Inport
  mi : Inport  Port=2
  z_m : Inport  Port=3
  x1 : Inport  Port=4
  x3 : Inport  Port=5
  y_2 : Inport  Port=6
  y4 : Inport  Port=7
  L : Inport  Port=8
  I_11 : Subsystem
  I_12 / I_21 : Subsystem
  I_13 / I_31_ : Subsystem
  I_22 : Subsystem
  I_23 / I_32 : Subsystem
  I_33 : Subsystem
  Mux : Mux  Inputs=9
  I_2_c : Outport
  wires:
  Mux/1 -> I_2_c/1  "PropSpeedCmd"
  m/1 -> I_12 / I_21/1(m), I_33/3(m), I_13 / I_31_/1(m), I_11/3(m), I_23 / I_32/1(m), I_22/3(m)
  mi/1 -> I_33/4(mi), I_13 / I_31_/2(mi), I_11/4(mi), I_23 / I_32/2(mi), I_12 / I_21/2(mi), I_22/4(mi)
  x1/1 -> I_33/6(x1), I_13 / I_31_/3(x1), I_22/1(x1), I_12 / I_21/5(x1)
  L/1 -> I_12 / I_21/7(L), I_11/6(L), I_23 / I_32/5(L), I_33/5(L)
  z_m/1 -> I_13 / I_31_/5(z_m), I_23 / I_32/6(z_m), I_11/5(z_m), I_22/5(z_m)
  y_2/1 -> I_11/1(y2), I_33/1(y2), I_23 / I_32/3(y2), I_12 / I_21/3(y2)
  y4/1 -> I_23 / I_32/4(y4), I_12 / I_21/4(y4), I_11/2(y4), I_33/2(y4)
  x3/1 -> I_33/7(x3), I_13 / I_31_/4(x3), I_22/2(x3), I_12 / I_21/6(x3)
  I_33/1(I_33) -> Mux/9
  I_11/1(I_11) -> Mux/1
  I_12 / I_21/1(I_12) -> Mux/4, Mux/2
  I_13 / I_31_/1(I_13) -> Mux/7, Mux/3
  I_22/1(I_22) -> Mux/5
  I_23 / I_32/1(I_23) -> Mux/8, Mux/6

== system MORUS_NELINEARNI_NELINEARNI_MPC_2/MORUS/I_3_c ==
  m : Inport
  mi : Inport  Port=2
  z_m : Inport  Port=3
  y2 : Inport  Port=4
  y4 : Inport  Port=5
  x1 : Inport  Port=6
  x3 : Inport  Port=7
  L : Inport  Port=8
  I_11 : Subsystem
  I_12 / I_21 : Subsystem
  I_13 / I_31 : Subsystem
  I_22 : Subsystem
  I_23 / I_32 : Subsystem
  I_33 : Subsystem
  Mux : Mux  Inputs=9
  I_3_c : Outport
  wires:
  I_11/1(I_11) -> Mux/1
  I_12 / I_21/1(I_12) -> Mux/2, Mux/4
  I_13 / I_31/1(I_13) -> Mux/3, Mux/7
  I_22/1(I_22) -> Mux/5
  I_23 / I_32/1(I_23) -> Mux/6, Mux/8
  I_33/1(I_33) -> Mux/9
  Mux/1 -> I_3_c/1  "PropSpeedCmd"
  m/1 -> I_12 / I_21/1(m), I_33/3(m), I_23 / I_32/1(m), I_22/3(m), I_13 / I_31/1(m), I_11/3(m)
  mi/1 -> I_33/4(mi), I_23 / I_32/2(mi), I_22/4(mi), I_13 / I_31/2(mi), I_12 / I_21/2(mi), I_11/4(mi)
  y2/1 -> I_33/6(y2), I_23 / I_32/3(y_2), I_11/1(y2), I_12 / I_21/5(y_2)
  L/1 -> I_12 / I_21/7(L), I_22/6(L), I_13 / I_31/5(L), I_33/5(L)
  z_m/1 -> I_23 / I_32/5(z_m), I_13 / I_31/6(z_m), I_22/5(z_m), I_11/5(z_m)
  x1/1 -> I_22/1(x1), I_33/1(x1), I_13 / I_31/3(x_1), I_12 / I_21/3(x_1)
  x3/1 -> I_13 / I_31/4(x_3), I_12 / I_21/4(x_3), I_22/2(x3), I_33/2(x3)
  y4/1 -> I_33/7(y4), I_23 / I_32/4(y_4), I_11/2(y4), I_12 / I_21/6(y_4)

== system MORUS_NELINEARNI_NELINEARNI_MPC_2/MORUS/I_4_c ==
  m : Inport
  mi : Inport  Port=2
  z_m : Inport  Port=3
  x_1 : Inport  Port=4
  x_3 : Inport  Port=5
  y2 : Inport  Port=6
  y4 : Inport  Port=7
  L : Inport  Port=8
  I_11 : Subsystem
  I_12 / I_21 : Subsystem
  I_13 / I_31_ : Subsystem
  I_22_ : Subsystem
  I_23 / I_32 : Subsystem
  I_33 : Subsystem
  Mux : Mux  Inputs=9
  I_4_c : Outport
  wires:
  I_12 / I_21/1(I_12) -> Mux/2, Mux/4
  I_23 / I_32/1(I_13) -> Mux/6, Mux/8
  I_33/1(I_33) -> Mux/9
  Mux/1 -> I_4_c/1  "PropSpeedCmd"
  m/1 -> I_12 / I_21/1(m), I_33/3(m), I_13 / I_31_/1(m), I_11/3(m), I_23 / I_32/1(m), I_22_/3(m)
  mi/1 -> I_33/4(mi), I_13 / I_31_/2(mi), I_11/4(mi), I_23 / I_32/2(mi), I_12 / I_21/2(mi), I_22_/4(mi)
  x_1/1 -> I_33/6(x_1), I_13 / I_31_/3(x1), I_22_/1(x1), I_12 / I_21/5(x1)
  L/1 -> I_12 / I_21/7(L), I_11/6(L), I_23 / I_32/5(L), I_33/5(L)
  z_m/1 -> I_13 / I_31_/5(z_m), I_23 / I_32/6(z_m), I_11/5(z_m), I_22_/5(z_m)
  y2/1 -> I_11/1(y2), I_33/1(y2), I_23 / I_32/3(y2), I_12 / I_21/3(y2)
  y4/1 -> I_23 / I_32/4(y4), I_12 / I_21/4(y4), I_11/2(y4), I_33/2(y4)
  x_3/1 -> I_33/7(x_3), I_13 / I_31_/4(x3), I_22_/2(x3), I_12 / I_21/6(x3)
  I_11/1(I_11) -> Mux/1
  I_22_/1(I_22) -> Mux/5
  I_13 / I_31_/1(I_13) -> Mux/7, Mux/3

== system MORUS_NELINEARNI_NELINEARNI_MPC_2/MORUS/I_b_c ==
  I_b_xx : Inport
  I_b_yy : Inport  Port=2
  I_b_zz : Inport  Port=3
  m_b : Inport  Port=4
  mi : Inport  Port=5
  z_m : Inport  Port=6
  y2 : Inport  Port=7
  y4 : Inport  Port=8
  x1 : Inport  Port=9
  x3 : Inport  Port=10
  I_11 : Subsystem
  I_12 / I_21 : Subsystem
  I_13 / I_31 : Subsystem
  I_22 : Subsystem
  I_23 / I_32 : Subsystem
  I_33 : Subsystem
  Mux : Mux  Inputs=9
  I_b_c : Outport
  wires:
  I_11/1(I_11) -> Mux/1
  I_12 / I_21/1(I_12) -> Mux/2, Mux/4
  I_13 / I_31/1(I_13) -> Mux/3, Mux/7
  I_22/1(I_22) -> Mux/5
  I_23 / I_32/1(I_23) -> Mux/6, Mux/8
  I_33/1(I_33) -> Mux/9
  Mux/1 -> I_b_c/1  "PropSpeedCmd"
  I_b_xx/1 -> I_11/1(I_b_xx)
  m_b/1 -> I_33/2(m_b), I_23 / I_32/1(m_b), I_22/2(m_b), I_13 / I_31/1(m_b), I_12 / I_21/1(m_b), I_11/2(m_b)
  I_b_yy/1 -> I_22/1(I_b_yy)
  I_b_zz/1 -> I_33/1(I_b_zz)
  mi/1 -> I_23 / I_32/2(mi), I_33/3(mi), I_22/3(mi), I_13 / I_31/2(mi), I_12 / I_21/2(mi), I_11/3(mi)
  z_m/1 -> I_23 / I_32/5(z_m), I_22/6(z_m), I_13 / I_31/5(z_m), I_11/6(z_m)
  y2/1 -> I_12 / I_21/5(y_2), I_23 / I_32/3(y_2), I_11/4(y2), I_33/4(y2)
  y4/1 -> I_23 / I_32/4(y_4), I_33/5(y4), I_11/5(y4), I_12 / I_21/6(y_4)
  x1/1 -> I_33/6(x1), I_13 / I_31/3(x_1), I_22/4(x_1), I_12 / I_21/3(x_1)
  x3/1 -> I_33/7(x3), I_13 / I_31/4(x_3), I_22/5(x_3), I_12 / I_21/4(x_3)

== system MORUS_NELINEARNI_NELINEARNI_MPC_2/MORUS/M_e_x ==
  M_r_1 : Inport
  M_r_3 : Inport  Port=2
  F_r_1 : Inport  Port=3
  F_r_2 : Inport  Port=4
  F_r_3 : Inport  Port=5
  F_r_4 : Inport  Port=6
  BETA : Inport  Port=7
  mi : Inport  Port=8
  z_m : Inport  Port=9
  y2 : Inport  Port=10
  y4 : Inport  Port=11
  L : Inport  Port=12
  z_r : Inport  Port=13
  Add : Sum  AccumDataTypeStr=double  OutDataTypeStr=double
  Add1 : Sum  Inputs=+-  AccumDataTypeStr=double  OutDataTypeStr=double
  Add2 : Sum  Inputs=-+  AccumDataTypeStr=double  OutDataTypeStr=double
  Add3 : Sum  Inputs=--  AccumDataTypeStr=double  OutDataTypeStr=double
  Add4 : Sum  Inputs=++++++++  AccumDataTypeStr=double  OutDataTypeStr=double
  Constant : Constant  Value=4  OutDataTypeStr=double  SampleTime=-1
  Cos : Trigonometry  Operator=cos
  Gain{,1..3} (4 alike) : Gain  Gain=-1
  Multiply : Product  Inputs=4
  Multiply{1,3,5,7} (4 alike) : Product
  Multiply2 : Product  Inputs=3
  Multiply4 : Product  Inputs=3
  Multiply6 : Product  Inputs=4
  Multiply8 : Product  Inputs=3
  Sin : Trigonometry
  M_e_x : Outport
  wires:
  BETA/1 -> Sin/1, Cos/1
  y2/1 -> Add/1
  y4/1 -> Add/2
  Gain/1 -> Multiply/1
  F_r_1/1 -> Gain/1
  Cos/1 -> Multiply8/2, Multiply2/2, Multiply6/2, Multiply/2
  mi/1 -> Multiply6/3, Multiply/3, Multiply4/1, Multiply3/1
  Add/1 -> Multiply3/2, Multiply6/4, Multiply/4  "errors"
  Gain1/1 -> Multiply1/1
  M_r_1/1 -> Gain1/1
  Sin/1 -> Multiply5/1, Multiply7/2, Multiply1/2
  F_r_2/1 -> Multiply2/1
  Add1/1 -> Multiply2/3  "errors"
  L/1 -> Add3/1, Add1/1
  Multiply3/1 -> Add3/2, Add1/2
  Constant/1 -> Multiply4/2
  z_m/1 -> Multiply4/3
  Multiply4/1 -> Add2/1
  z_r/1 -> Add2/2
  Add2/1 -> Multiply5/2  "errors"
  Gain2/1 -> Multiply6/1
  F_r_3/1 -> Gain2/1
  M_r_3/1 -> Multiply7/1
  Add3/1 -> Multiply8/3  "errors"
  F_r_4/1 -> Multiply8/1
  Multiply1/1 -> Add4/1
  Multiply7/1 -> Add4/2
  Multiply8/1 -> Add4/3
  Multiply2/1 -> Add4/4
  Multiply6/1 -> Add4/5
  Multiply/1 -> Add4/6
  Multiply5/1 -> Add4/7, Gain3/1
  Gain3/1 -> Add4/8
  Add4/1 -> M_e_x/1  "errors"

== system MORUS_NELINEARNI_NELINEARNI_MPC_2/MORUS/M_e_y ==
  M_r_4 : Inport
  M_r_2 : Inport  Port=2
  F_r2 : Inport  Port=3
  F_r3 : Inport  Port=4
  F_r4 : Inport  Port=5
  F_r1 : Inport  Port=6
  BETA : Inport  Port=7
  mi : Inport  Port=8
  z_m : Inport  Port=9
  x1 : Inport  Port=10
  x3 : Inport  Port=11
  L : Inport  Port=12
  z_r : Inport  Port=13
  Add : Sum  AccumDataTypeStr=double  OutDataTypeStr=double
  Add1 : Sum  AccumDataTypeStr=double  OutDataTypeStr=double
  Add2 : Sum  Inputs=-+  AccumDataTypeStr=double  OutDataTypeStr=double
  Add3 : Sum  Inputs=-+  AccumDataTypeStr=double  OutDataTypeStr=double
  Add4 : Sum  Inputs=++++++++  AccumDataTypeStr=double  OutDataTypeStr=double
  Constant : Constant  Value=4  OutDataTypeStr=double  SampleTime=-1
  Cos : Trigonometry  Operator=cos
  Gain1 : Gain  Gain=-1
  Gain3 : Gain  Gain=-1
  Multiply : Product  Inputs=4
  Multiply{1,3,5,7} (4 alike) : Product
  Multiply2 : Product  Inputs=3
  Multiply4 : Product  Inputs=3
  Multiply6 : Product  Inputs=4
  Multiply8 : Product  Inputs=3
  Sin : Trigonometry
  M_e_y : Outport
  wires:
  BETA/1 -> Sin/1, Cos/1
  x1/1 -> Add/1
  x3/1 -> Add/2
  F_r2/1 -> Multiply/1
  Cos/1 -> Multiply8/2, Multiply2/2, Multiply6/2, Multiply/2
  mi/1 -> Multiply6/3, Multiply/3, Multiply4/1, Multiply3/1
  Add/1 -> Multiply3/2, Multiply6/4, Multiply/4  "errors"
  Gain1/1 -> Multiply1/1
  M_r_4/1 -> Gain1/1
  Sin/1 -> Multiply5/1, Multiply7/2, Multiply1/2
  F_r3/1 -> Multiply2/1
  Add1/1 -> Multiply2/3  "errors"
  L/1 -> Add3/1, Add1/1
  Multiply3/1 -> Add3/2, Add1/2
  Constant/1 -> Multiply4/2
  z_m/1 -> Multiply4/3
  Multiply4/1 -> Add2/1
  z_r/1 -> Add2/2
  Add2/1 -> Multiply5/2  "errors"
  F_r4/1 -> Multiply6/1
  M_r_2/1 -> Multiply7/1
  Add3/1 -> Multiply8/3  "errors"
  F_r1/1 -> Multiply8/1
  Multiply1/1 -> Add4/1
  Multiply7/1 -> Add4/2
  Multiply8/1 -> Add4/3
  Multiply2/1 -> Add4/4
  Multiply6/1 -> Add4/5
  Multiply/1 -> Add4/6
  Multiply5/1 -> Add4/7, Gain3/1
  Gain3/1 -> Add4/8
  Add4/1 -> M_e_y/1  "errors"

== system MORUS_NELINEARNI_NELINEARNI_MPC_2/MORUS/M_e_z ==
  F_r_1 : Inport
  F_r_2 : Inport  Port=2
  F_r_3 : Inport  Port=3
  F_r_4 : Inport  Port=4
  M_r_1 : Inport  Port=5
  M_r_2 : Inport  Port=6
  M_r_3 : Inport  Port=7
  M_r_4 : Inport  Port=8
  BETA : Inport  Port=9
  x1 : Inport  Port=10
  x3 : Inport  Port=11
  y2 : Inport  Port=12
  y4 : Inport  Port=13
  mi : Inport  Port=14
  Add : Sum  AccumDataTypeStr=double  OutDataTypeStr=double
  Add1 : Sum  AccumDataTypeStr=double  OutDataTypeStr=double
  Add2 : Sum  Inputs=++++++++  AccumDataTypeStr=double  OutDataTypeStr=double
  Cos : Trigonometry  Operator=cos
  Gain{,1..3} (4 alike) : Gain  Gain=-1
  Multiply{,1..3} (4 alike) : Product
  Multiply{4..7} (4 alike) : Product  Inputs=4
  Sin : Trigonometry
  M_e_z : Outport
  wires:
  x1/1 -> Add/1
  x3/1 -> Add/2
  y2/1 -> Add1/1
  y4/1 -> Add1/2
  BETA/1 -> Sin/1, Cos/1
  Cos/1 -> Multiply/2, Multiply1/2, Multiply2/2, Multiply3/2
  Gain/1 -> Multiply1/1
  Gain1/1 -> Multiply3/1
  M_r_4/1 -> Gain1/1
  M_r_2/1 -> Gain/1
  M_r_3/1 -> Multiply2/1
  M_r_1/1 -> Multiply/1
  Gain2/1 -> Multiply7/1
  F_r_4/1 -> Gain2/1
  Gain3/1 -> Multiply4/1
  F_r_1/1 -> Gain3/1
  F_r_2/1 -> Multiply5/1
  F_r_3/1 -> Multiply6/1
  Sin/1 -> Multiply6/2, Multiply4/2, Multiply5/2, Multiply7/2
  mi/1 -> Multiply6/3, Multiply5/3, Multiply4/3, Multiply7/3
  Add/1 -> Multiply7/4, Multiply5/4  "errors"
  Add1/1 -> Multiply6/4, Multiply4/4  "errors"
  Add2/1 -> M_e_z/1  "errors"
  Multiply4/1 -> Add2/1
  Multiply5/1 -> Add2/2
  Multiply6/1 -> Add2/3
  Multiply7/1 -> Add2/4
  Multiply/1 -> Add2/5
  Multiply1/1 -> Add2/6
  Multiply2/1 -> Add2/7
  Multiply3/1 -> Add2/8

== system MORUS_NELINEARNI_NELINEARNI_MPC_2/MORUS/Moment rotor 1 ==
  Force_1 : Inport
  b_m : Inport  Port=2
  zeta_1 : Inport  Port=3
  Multiply : Product  Inputs=3  OutDataTypeStr=double
  Moment_1 : Outport
  wires:
  Multiply/1 -> Moment_1/1
  b_m/1 -> Multiply/2
  Force_1/1 -> Multiply/1
  zeta_1/1 -> Multiply/3

== system MORUS_NELINEARNI_NELINEARNI_MPC_2/MORUS/Moment rotor 2 ==
  Force_2 : Inport
  b_m : Inport  Port=2
  zeta_2 : Inport  Port=3
  Multiply : Product  Inputs=3  OutDataTypeStr=double
  Moment_2 : Outport
  wires:
  Multiply/1 -> Moment_2/1
  b_m/1 -> Multiply/2
  Force_2/1 -> Multiply/1
  zeta_2/1 -> Multiply/3

== system MORUS_NELINEARNI_NELINEARNI_MPC_2/MORUS/Moment rotor 3 ==
  Force_3 : Inport
  b_m : Inport  Port=2
  zeta_3 : Inport  Port=3
  Multiply : Product  Inputs=3  OutDataTypeStr=double
  Moment_3 : Outport
  wires:
  Multiply/1 -> Moment_3/1
  b_m/1 -> Multiply/2
  Force_3/1 -> Multiply/1
  zeta_3/1 -> Multiply/3

== system MORUS_NELINEARNI_NELINEARNI_MPC_2/MORUS/Moment rotor 4 ==
  Force_4 : Inport
  b_m : Inport  Port=2
  zeta_4 : Inport  Port=3
  Multiply : Product  Inputs=3  OutDataTypeStr=double
  Moment_4 : Outport
  wires:
  Multiply/1 -> Moment_4/1
  b_m/1 -> Multiply/2
  Force_4/1 -> Multiply/1
  zeta_4/1 -> Multiply/3

== system MORUS_NELINEARNI_NELINEARNI_MPC_2/MORUS/SERVO MASA 1 ==
  ref_masa_1 : Inport  OutDataTypeStr=double
  Derivative : Derivative
  Derivative1 : Derivative
  Scope : Scope
  Transfer Fcn : TransferFcn  Numerator=[w_mm^2]  Denominator=[1 2*zeta_mm*w_mm w_mm^2]
  masa_1/x1 : Outport  OutDataTypeStr=double
  "dot_x_1 " : Outport  Port=2
  "dot_dot_x_1 " : Outport  Port=3
  wires:
  ref_masa_1/1 -> Transfer Fcn/1
  Derivative1/1 -> Scope/1, "dot_dot_x_1 "/1  "errors"
  Derivative/1 -> Derivative1/1, "dot_x_1 "/1
  Transfer Fcn/1 -> Derivative/1, masa_1/x1/1

== system MORUS_NELINEARNI_NELINEARNI_MPC_2/MORUS/SERVO MASA 2 ==
  ref_masa_2 : Inport
  Constant : Constant  Value=0  OutDataTypeStr=double  SampleTime=-1
  Derivative : Derivative
  Derivative1 : Derivative
  Sum : Sum  Inputs=|++
  Transfer Fcn : TransferFcn  Numerator=[w_mm^2]  Denominator=[1 2*zeta_mm*w_mm w_mm^2]
  masa_2/y2 : Outport
  "dot_y_2 " : Outport  Port=2
  "dot_dot_y_2 " : Outport  Port=3
  wires:
  ref_masa_2/1 -> Transfer Fcn/1
  Sum/1 -> Derivative/1, masa_2/y2/1
  Derivative1/1 -> "dot_dot_y_2 "/1  "errors"
  Constant/1 -> Sum/2
  Transfer Fcn/1 -> Sum/1
  Derivative/1 -> Derivative1/1, "dot_y_2 "/1

== system MORUS_NELINEARNI_NELINEARNI_MPC_2/MORUS/SERVO MASA 3 ==
  ref_masa_3 : Inport
  Constant : Constant  Value=0  OutDataTypeStr=double  SampleTime=-1
  Derivative : Derivative
  Derivative1 : Derivative
  Gain : Gain  Gain=0
  Step : Step  After=0.01  SampleTime=0
  Step1 : Step  Time=1.1  After=-0.01  SampleTime=0
  Sum : Sum  Inputs=|+++
  Sum1 : Sum  Inputs=|++
  Transfer Fcn : TransferFcn  Numerator=[w_mm^2]  Denominator=[1 2*zeta_mm*w_mm w_mm^2]
  masa_3/x3 : Outport
  "dot_x_3 " : Outport  Port=2
  "dot_dot_x_3 " : Outport  Port=3
  wires:
  ref_masa_3/1 -> Transfer Fcn/1
  Sum/1 -> Derivative/1, masa_3/x3/1
  Derivative1/1 -> "dot_dot_x_3 "/1  "errors"
  Constant/1 -> Sum/2
  Transfer Fcn/1 -> Sum/1
  Step1/1 -> Sum1/2
  Step/1 -> Sum1/1
  Sum1/1 -> Gain/1
  Gain/1 -> Sum/3
  Derivative/1 -> Derivative1/1, "dot_x_3 "/1

== system MORUS_NELINEARNI_NELINEARNI_MPC_2/MORUS/SERVO MASA 4 ==
  ref_masa_4 : Inport
  Constant : Constant  Value=0  OutDataTypeStr=double  SampleTime=-1
  Derivative : Derivative
  Derivative1 : Derivative
  Sum : Sum  Inputs=|++
  Transfer Fcn : TransferFcn  Numerator=[w_mm^2]  Denominator=[1 2*zeta_mm*w_mm w_mm^2]
  masa_4/y4 : Outport
  "dot_y_4 " : Outport  Port=2
  "dot_dot_y_4 " : Outport  Port=3
  wires:
  ref_masa_4/1 -> Transfer Fcn/1
  Sum/1 -> Derivative/1, masa_4/y4/1
  Constant/1 -> Sum/2
  Transfer Fcn/1 -> Sum/1
  Derivative/1 -> Derivative1/1, "dot_y_4 "/1
  Derivative1/1 -> "dot_dot_y_4 "/1

== system MORUS_NELINEARNI_NELINEARNI_MPC_2/MORUS/Subsystem1 ==
  "DOT_W_X " : Inport
  Integrator : Integrator
  W_X : Outport
  wires:
  "DOT_W_X "/1 -> Integrator/1
  Integrator/1 -> W_X/1

== system MORUS_NELINEARNI_NELINEARNI_MPC_2/MORUS/Subsystem2 ==
  "DOT_W_Y " : Inport
  Integrator : Integrator
  W_Y : Outport
  wires:
  "DOT_W_Y "/1 -> Integrator/1
  Integrator/1 -> W_Y/1

== system MORUS_NELINEARNI_NELINEARNI_MPC_2/MORUS/Subsystem3 ==
  "DOT_W_Z " : Inport
  Integrator : Integrator
  W_Z : Outport
  wires:
  "DOT_W_Z "/1 -> Integrator/1
  Integrator/1 -> W_Z/1

== system MORUS_NELINEARNI_NELINEARNI_MPC_2/MORUS/Subsystem4 ==
  "DOT_ROLL " : Inport
  Integrator : Integrator
  ROLL : Outport
  wires:
  "DOT_ROLL "/1 -> Integrator/1
  Integrator/1 -> ROLL/1

== system MORUS_NELINEARNI_NELINEARNI_MPC_2/MORUS/Subsystem5 ==
  "DOT_PITCH " : Inport
  Integrator : Integrator
  PITCH : Outport
  wires:
  "DOT_PITCH "/1 -> Integrator/1
  Integrator/1 -> PITCH/1

== system MORUS_NELINEARNI_NELINEARNI_MPC_2/MORUS/Subsystem6 ==
  "DOT_YAW " : Inport
  Integrator : Integrator
  YAW : Outport
  wires:
  "DOT_YAW "/1 -> Integrator/1
  Integrator/1 -> YAW/1

== system MORUS_NELINEARNI_NELINEARNI_MPC_2/MORUS/Subsystem7 ==
  "DOT_DOT_Y " : Inport
  Gain : Gain  Gain=0.5*1.24*1*2
  Integrator : Integrator
  Integrator1 : Integrator
  Product : Product
  Sign : Signum
  Square : Math  Operator=square  SaturateOnIntegerOverflow=on
  Sum : Sum  Inputs=|+-
  Y : Outport
  DOT_Y : Outport  Port=2
  wires:
  "DOT_DOT_Y "/1 -> Sum/1
  Integrator/1 -> Sign/1, DOT_Y/1, Integrator1/1, Square/1
  Integrator1/1 -> Y/1
  Sum/1 -> Integrator/1
  Product/1 -> Sum/2
  Gain/1 -> Product/2
  Sign/1 -> Gain/1
  Square/1 -> Product/1

== system MORUS_NELINEARNI_NELINEARNI_MPC_2/MORUS/Subsystem8 ==
  "DOT_DOT_X " : Inport
  Gain : Gain  Gain=0.5*1.24*1*2
  Integrator : Integrator
  Integrator1 : Integrator
  Product : Product
  Sign : Signum
  Square : Math  Operator=square  SaturateOnIntegerOverflow=on
  Sum : Sum  Inputs=|+-
  X : Outport
  DOT_X : Outport  Port=2
  wires:
  "DOT_DOT_X "/1 -> Sum/1
  Integrator1/1 -> X/1
  Square/1 -> Product/1
  Integrator/1 -> Square/1, DOT_X/1, Sign/1, Integrator1/1
  Sign/1 -> Gain/1
  Product/1 -> Sum/2
  Gain/1 -> Product/2
  Sum/1 -> Integrator/1

== system MORUS_NELINEARNI_NELINEARNI_MPC_2/MORUS/Subsystem9 ==
  "DOT_DOT_Z " : Inport
  Gain : Gain  Gain=0.5*1.24*1*2
  Integrator : Integrator
  Integrator1 : Integrator
  Product : Product
  Saturation : Saturate  UpperLimit=250  LowerLimit=0  OutDataTypeStr=double
      settings: AttributesFormatString=%<LowerLimit>\nto\n%<UpperLimit>
  Sign : Signum
  Square : Math  Operator=square  SaturateOnIntegerOverflow=on
  Sum : Sum  Inputs=|+-
  Z : Outport
  DOT_Z : Outport  Port=2
  wires:
  "DOT_DOT_Z "/1 -> Sum/1
  Integrator1/1 -> Saturation/1
  Saturation/1 -> Z/1
  Square/1 -> Product/1
  Integrator/1 -> Sign/1, DOT_Z/1, Integrator1/1, Square/1
  Sign/1 -> Gain/1
  Product/1 -> Sum/2
  Gain/1 -> Product/2
  Sum/1 -> Integrator/1

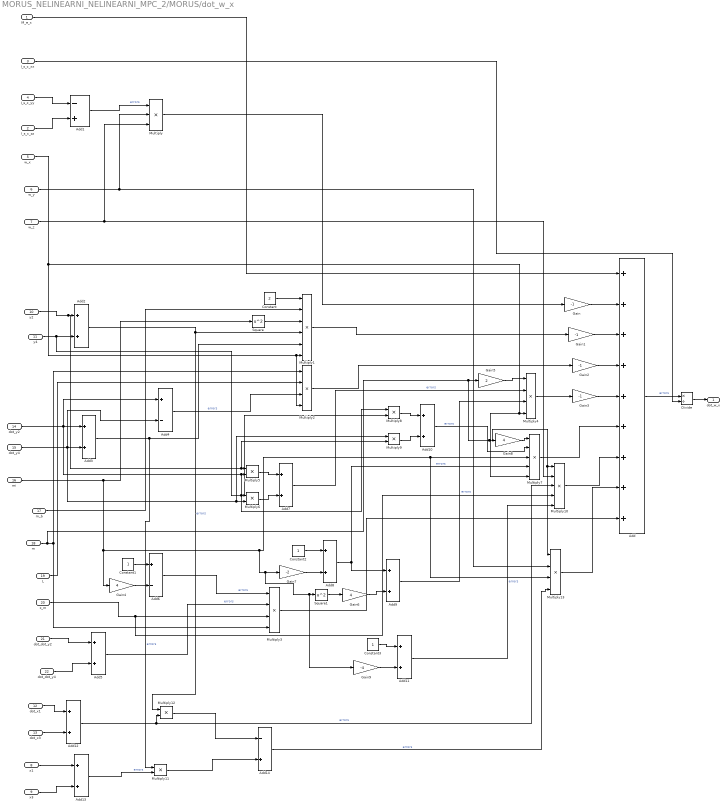
== system MORUS_NELINEARNI_NELINEARNI_MPC_2/MORUS/dot_w_x ==
  M_e_x : Inport
  I_s_c_zz : Inport  Port=2
  I_s_c_xx : Inport  Port=3
  I_s_c_yy : Inport  Port=4
  w_x : Inport  Port=5
  w_y : Inport  Port=6
  w_z : Inport  Port=7
  x1 : Inport  Port=8
  x3 : Inport  Port=9
  y2 : Inport  Port=10
  y4 : Inport  Port=11
  dot_x1 : Inport  Port=12
  dot_x3 : Inport  Port=13
  dot_y2 : Inport  Port=14
  dot_y4 : Inport  Port=15
  mi : Inport  Port=16
  m_b : Inport  Port=17
  m : Inport  Port=18
  L : Inport  Port=19
  z_m : Inport  Port=20
  dot_dot_y2 : Inport  Port=21
  dot_dot_y4 : Inport  Port=22
  Add : Sum  Inputs=+++++++++  AccumDataTypeStr=double  OutDataTypeStr=double
  Add1 : Sum  Inputs=-+  AccumDataTypeStr=double  OutDataTypeStr=double
  Add{2..3,5,7..13} (10 alike) : Sum  AccumDataTypeStr=double  OutDataTypeStr=double
  Add14 : Sum  Inputs=-+  AccumDataTypeStr=double  OutDataTypeStr=double
  Add4 : Sum  Inputs=+-  AccumDataTypeStr=double  OutDataTypeStr=double
  Add6 : Sum  Inputs=+-  AccumDataTypeStr=double  OutDataTypeStr=double
  Constant : Constant  Value=2  OutDataTypeStr=double  SampleTime=-1
  Constant1 : Constant  OutDataTypeStr=double  SampleTime=-1
  Constant2 : Constant  OutDataTypeStr=double  SampleTime=-1
  Constant3 : Constant  OutDataTypeStr=double  SampleTime=-1
  Divide : Product  Inputs=*/
  Gain{,1..3} (4 alike) : Gain  Gain=-1
  Gain4 : Gain  Gain=4
  Gain5 : Gain  Gain=2
  Gain6 : Gain  Gain=4
  Gain7 : Gain  Gain=-2
  Gain8 : Gain  Gain=4
  Gain9 : Gain  Gain=-4
  Multiply : Product  Inputs=3
  Multiply1 : Product  Inputs=6
  Multiply10 : Product  Inputs=5
  Multiply{5..6,8..9,11..12} (6 alike) : Product
  Multiply{2..4,13} (4 alike) : Product  Inputs=4
  Multiply7 : Product  Inputs=5
  Square : Math  Operator=square  SaturateOnIntegerOverflow=on
  Square1 : Math  Operator=square  SaturateOnIntegerOverflow=on
  dot_w_x : Outport
  wires:
  Add/1 -> Divide/1  "errors"
  I_s_c_xx/1 -> Divide/2
  Divide/1 -> dot_w_x/1
  M_e_x/1 -> Add/1
  Gain/1 -> Add/2
  Gain1/1 -> Add/3
  Gain2/1 -> Add/4
  Gain3/1 -> Add/5
  I_s_c_zz/1 -> Add1/2
  I_s_c_yy/1 -> Add1/1
  Add1/1 -> Multiply/1  "errors"
  w_y/1 -> Multiply13/2, Multiply/2
  w_z/1 -> Multiply10/2, Multiply/3
  Multiply/1 -> Gain/1
  y2/1 -> Multiply9/2, Multiply5/1, Add2/1
  y4/1 -> Multiply8/2, Multiply6/1, Add2/2
  dot_y2/1 -> Add4/1, Add3/1, Multiply8/1, Multiply5/2
  dot_y4/1 -> Add4/2, Add3/2, Multiply6/2, Multiply9/1
  Multiply1/1 -> Gain1/1
  Add2/1 -> Multiply12/1, Multiply1/4  "errors"
  Add3/1 -> Multiply11/1, Multiply1/5  "errors"
  w_x/1 -> Multiply4/4, Multiply7/5, Multiply2/4, Multiply1/6
  Constant/1 -> Multiply1/1
  m_b/1 -> Multiply1/2
  Square/1 -> Multiply1/3
  mi/1 -> Gain4/1, Multiply13/3, Multiply7/3, Gain9/1, Square1/1, Gain7/1, Square/1
  Multiply2/1 -> Gain2/1
  Add4/1 -> Multiply2/3  "errors"
  L/1 -> Multiply2/2
  dot_dot_y4/1 -> Add5/2
  dot_dot_y2/1 -> Add5/1
  Gain4/1 -> Add6/2
  Constant1/1 -> Add6/1
  Add6/1 -> Multiply3/1  "errors"
  Add5/1 -> Multiply3/2  "errors"
  z_m/1 -> Multiply10/4, Multiply3/3
  Multiply3/1 -> Add/9
  Multiply4/1 -> Gain3/1
  Gain5/1 -> Multiply4/1
  m/1 -> Multiply13/1, Multiply10/1, Gain8/1, Gain5/1, Multiply3/4, Multiply2/1
  Multiply5/1 -> Add7/1
  Multiply6/1 -> Add7/2
  Add7/1 -> Multiply4/2  "errors"
  Add8/1 -> Add9/1, Multiply7/4  "errors"
  Gain6/1 -> Add9/2
  Gain7/1 -> Add8/2
  Square1/1 -> Gain6/1
  Add9/1 -> Multiply4/3  "errors"
  Constant2/1 -> Add8/1
  Gain8/1 -> Multiply7/1
  Multiply9/1 -> Add10/2
  Multiply8/1 -> Add10/1
  Add10/1 -> Multiply7/2  "errors"
  Multiply7/1 -> Add/6
  Gain9/1 -> Add11/2
  Constant3/1 -> Add11/1
  Multiply10/1 -> Add/7
  dot_x1/1 -> Add12/1
  dot_x3/1 -> Add12/2
  Add11/1 -> Multiply10/5  "errors"
  Add12/1 -> Multiply12/2, Multiply10/3  "errors"
  x1/1 -> Add13/1
  x3/1 -> Add13/2
  Add13/1 -> Multiply11/2  "errors"
  Multiply11/1 -> Add14/2
  Multiply12/1 -> Add14/1
  Multiply13/1 -> Add/8
  Add14/1 -> Multiply13/4  "errors"
